simulink model "fpid0"  (R2016a)
settings: Solver=VariableStepAuto  StartTime=0.0  StopTime=5  MaxStep=0.01  RelTol=1e-4
values from neighbouring files (symbols this model uses):
  GCE = GE*(kp-imag(sqrt(kp*kp-4*ki*kd)))/2/ki    [update_gains0.m]
  GCU = ki/GE    [update_gains0.m]
  GE = 10    [fpidinit.mat]
  GU = kd/GCE    [update_gains0.m]
  kd = 0.02    [fpidinit.mat]
  ki = 22    [fpidinit.mat]
  kp = 1.2    [fpidinit.mat]
libraries: fuzblock x1, simulink x1
settings Model: Creator=jcjqyb  LastModifiedBy=zy5f9
settings DataIOCC: LimitDataPoints=on  SaveOutput=off  SaveTime=off
settings OptimizationCC: ExpressionDepthLimit=2147483647  LifeSpan=1
settings DebuggingCC: UnderspecifiedInitializationDetection=Classic  MergeDetectMultiDrivingBlocksExec=none  FcnCallInpInsideContextMsg=EnableAllAsWarning  AllowSymbolicDim=off  StateNameClashWarn=warning
settings GRTTargetCC: CombineOutputUpdateFcns=off  GRTInterface=on

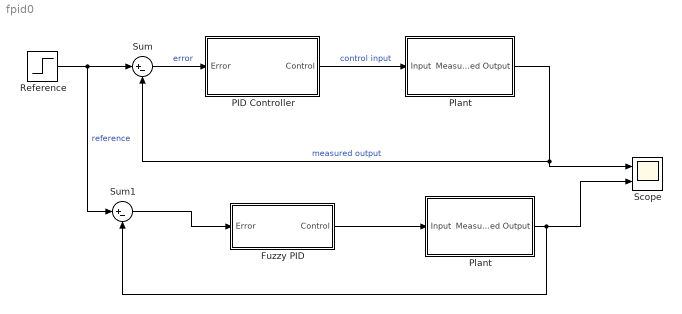
== system fpid0 ==
  Fuzzy PID : Subsystem
  PID Controller : Subsystem
  Plant : Subsystem
  "Plant " : Subsystem
  Reference : Step  SampleTime=0
  Scope : Scope  NumInputPorts=2
  Sum : Sum  Inputs=|+-
  Sum1 : Sum  Inputs=|+-
  wires:
  Reference/1 -> Sum1/1, Sum/1  "reference"
  Plant/1(Measured Output) -> Scope/1, Sum/2  "measured output"
  Sum/1 -> PID Controller/1(Error)  "error"
  PID Controller/1(Control) -> Plant/1(Input)  "control input"
  Sum1/1 -> Fuzzy PID/1(Error)
  Fuzzy PID/1(Control) -> "Plant "/1(Input)
  "Plant "/1(Measured Output) -> Scope/2, Sum1/2

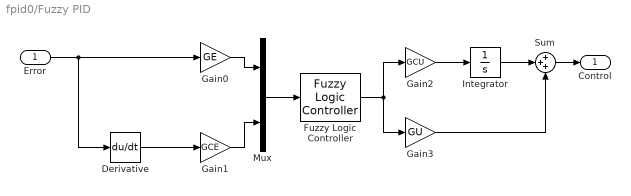
== system fpid0/Fuzzy PID ==
  Error : Inport
  Derivative : Derivative
  Fuzzy Logic Controller : fuzblock/Fuzzy Logic  Controller  fis=FIS
  Gain0 : Gain  Gain=GE
  Gain1 : Gain  Gain=GCE
  Gain2 : Gain  Gain=GCU
  Gain3 : Gain  Gain=GU
  Integrator : Integrator
  Mux : Mux  Inputs=2
  Sum : Sum  Inputs=+++
  Control : Outport
  wires:
  Error/1 -> Derivative/1, Gain0/1
  Mux/1 -> Fuzzy Logic Controller/1
  Gain0/1 -> Mux/1
  Gain1/1 -> Mux/2
  Fuzzy Logic Controller/1 -> Gain3/1, Gain2/1
  Gain3/1 -> Sum/3
  Sum/1 -> Control/1
  Derivative/1 -> Gain1/1
  Integrator/1 -> Sum/2
  Gain2/1 -> Integrator/1

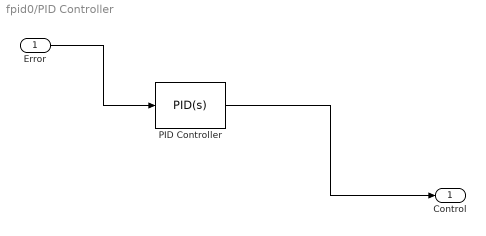
== system fpid0/PID Controller ==
  Error : Inport
  PID Controller : simulink/Continuous/PID Controller  Controller=PID  TimeDomain=Continuous-time  SampleTime=-1  IntegratorMethod=Forward Euler  FilterMethod=Forward Euler  Form=Parallel  UseFilter=on  ControllerParametersSource=internal  P=kp  I=ki  D=kd  N=20  InitialConditionSource=internal  InitialConditionForIntegrator=0  InitialConditionForFilter=0  ExternalReset=none  LimitOutput=off  UpperSaturationLimit=inf  LowerSaturationLimit=-inf  LinearizeAsGain=on  AntiWindupMode=none  Kb=1  TrackingMode=off  Kt=1  PParamMin=[]  PParamMax=[]  IParamMin=[]  IParamMax=[]  DParamMin=[]  DParamMax=[]  NParamMin=[]  NParamMax=[]  KbParamMin=[]  KbParamMax=[]  KtParamMin=[]  KtParamMax=[]  POutMin=[]  POutMax=[]  IOutMin=[]  IOutMax=[]  DOutMin=[]  DOutMax=[]  NOutMin=[]  NOutMax=[]  KbOutMin=[]  KbOutMax=[]  KtOutMin=[]  KtOutMax=[]  IntegratorOutMin=[]  IntegratorOutMax=[]  FilterOutMin=[]  FilterOutMax=[]  SumOutMin=[]  SumOutMax=[]  SumI1OutMin=[]  SumI1OutMax=[]  SumI2OutMin=[]  SumI2OutMax=[]  SumI3OutMin=[]  SumI3OutMax=[]  SumDOutMin=[]  SumDOutMax=[]  SaturationOutMin=[]  SaturationOutMax=[]  IntegratorContinuousStateAttributes=''  IntegratorStateMustResolveToSignalObject=off  IntegratorRTWStateStorageClass=Auto  FilterContinuousStateAttributes=''  FilterStateMustResolveToSignalObject=off  FilterRTWStateStorageClass=Auto  DifferentiatorICPrevScaledInput=0  DifferentiatorOutMin=[]  DifferentiatorOutMax=[]
  Control : Outport
  wires:
  Error/1 -> PID Controller/1
  PID Controller/1 -> Control/1

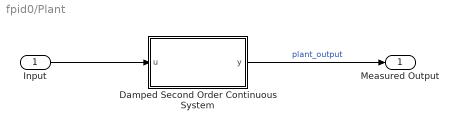
== system fpid0/Plant ==
  Input : Inport
  Damped Second Order Continuous System : Subsystem  mask{wn=16, zeta=0.6}
      mask prompts: wn "Undamped natural frequency (wn, rad/s)"; zeta "Damping factor (zeta)"
  Measured Output : Outport
  wires:
  Input/1 -> Damped Second Order Continuous System/1(u)
  Damped Second Order Continuous System/1(y) -> Measured Output/1  "plant_output"

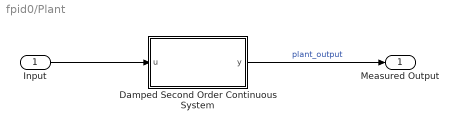
== system fpid0/Plant  ==
  Input : Inport
  Damped Second Order Continuous System : Subsystem  mask{wn=16, zeta=0.6}
      mask prompts: wn "Undamped natural frequency (wn, rad/s)"; zeta "Damping factor (zeta)"
  Measured Output : Outport
  wires:
  Input/1 -> Damped Second Order Continuous System/1(u)
  Damped Second Order Continuous System/1(y) -> Measured Output/1  "plant_output"

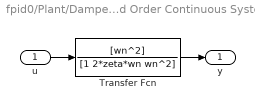
== system fpid0/Plant/Damped Second Order Continuous System ==
  u : Inport
  Transfer Fcn : TransferFcn  Numerator=[wn^2]  Denominator=[1 2*zeta*wn wn^2]
  y : Outport
  wires:
  Transfer Fcn/1 -> y/1
  u/1 -> Transfer Fcn/1

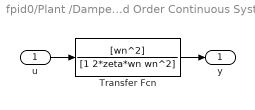
== system fpid0/Plant /Damped Second Order Continuous System ==
  u : Inport
  Transfer Fcn : TransferFcn  Numerator=[wn^2]  Denominator=[1 2*zeta*wn wn^2]
  y : Outport
  wires:
  Transfer Fcn/1 -> y/1
  u/1 -> Transfer Fcn/1
